simulink model "RCAM_simulation"  (R2021a)
settings: Solver=VariableStepAuto  StartTime=0.0  StopTime=200  RelTol=1e-3
values from neighbouring files (symbols this model uses):
  x0 = [85;0;0;0;0;0;0;0.1;0]    [init.m]
undefined symbols (not defined in the file or in its folder): RCAM_model
settings Model: Creator=Chitra Manis Raja  LastModifiedBy=Chitra Manis Raja

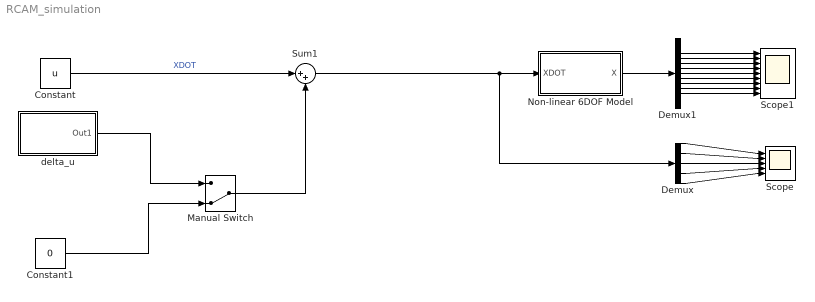
== system RCAM_simulation ==
  Constant : Constant  Value=u
  Constant1 : Constant  Value=0
  Demux : Demux  Outputs=5
  Demux1 : Demux  Outputs=9
  Manual Switch : ManualSwitch  CurrentSetting=0
  Non-linear 6DOF Model : Subsystem
  Scope : Scope  NumInputPorts=5
  Scope1 : Scope  NumInputPorts=9
  Sum1 : Sum  Inputs=|++
  delta_u : Subsystem
  wires:
  Non-linear 6DOF Model/1(X) -> Demux1/1
  Constant/1 -> Sum1/1  "XDOT"
  Sum1/1 -> Non-linear 6DOF Model/1(XDOT), Demux/1
  Demux/1 -> Scope/1
  Demux/2 -> Scope/2
  Demux/3 -> Scope/3
  Demux/4 -> Scope/4
  Demux/5 -> Scope/5
  Demux1/1 -> Scope1/1
  Demux1/2 -> Scope1/2
  Demux1/3 -> Scope1/3
  Demux1/4 -> Scope1/4
  Demux1/5 -> Scope1/5
  Demux1/6 -> Scope1/6
  Demux1/7 -> Scope1/7
  Demux1/8 -> Scope1/8
  Demux1/9 -> Scope1/9
  Manual Switch/1 -> Sum1/2
  delta_u/1(Out1) -> Manual Switch/1
  Constant1/1 -> Manual Switch/2

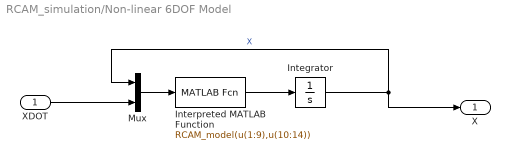
== system RCAM_simulation/Non-linear 6DOF Model ==
  XDOT : Inport
  Integrator : Integrator  InitialCondition=x0
  Interpreted MATLAB Function : MATLABFcn  MATLABFcn=RCAM_model(u(1:9),u(10:14))
  Mux : Mux  Inputs=2
  X : Outport
  wires:
  Integrator/1 -> X/1, Mux/1  "X"
  Mux/1 -> Interpreted MATLAB Function/1
  Interpreted MATLAB Function/1 -> Integrator/1
  XDOT/1 -> Mux/2

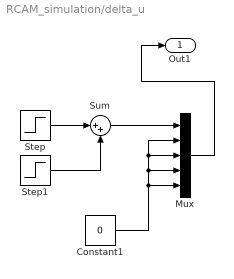
== system RCAM_simulation/delta_u ==
  Constant1 : Constant  Value=0
  Mux : Mux  Inputs=5
  Step : Step  Time=30  After=5*pi/180  SampleTime=0
  Step1 : Step  Time=30+2  After=-5*pi/180  SampleTime=0
  Sum : Sum  Inputs=|++
  Out1 : Outport
  wires:
  Sum/1 -> Mux/1
  Constant1/1 -> Mux/5, Mux/4, Mux/2, Mux/3
  Step1/1 -> Sum/2
  Step/1 -> Sum/1
  Mux/1 -> Out1/1
